simulink model "mainModel"  (R2024b)
settings: Solver=ode4  StartTime=0.0  StopTime=35000  FixedStep=0.1  RelTol=1e-3
values from neighbouring files (symbols this model uses):
  actuators = actuatorsConfig()    [main.m]
  constant = constantsConfig()    [main.m]
  control = controlConfig(data)    [main.m]
  MEKF = estimationConfig(sensors,simOpt)    [main.m]
  pert = pertConfig()    [main.m]
  sensors = sensorsConfig()    [main.m]
undefined symbols (not defined in the file or in its folder): Ab0, data, DiscIntNeverNeededParam, init
libraries: matrix_library x38, simulink x10, aerolibutil x7, simulink_extras x6, sharedtransform x1, dspinverses x1, dspfdesign x1, dspstat3 x1
(part 1 of 3)
settings Model: SimulationMode=accelerator  Creator=ricca  LastModifiedBy=ricca

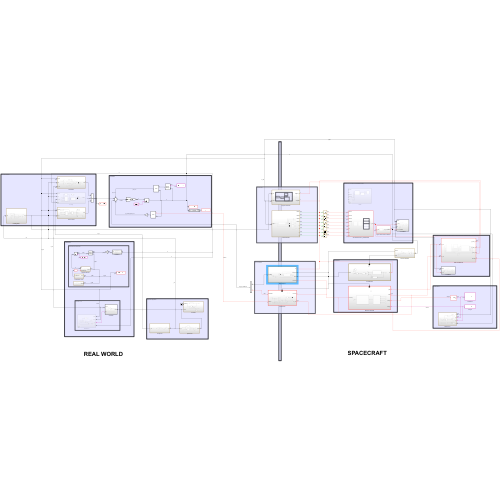
[thumbnail: Simulink's stored preview of the top-level diagram]
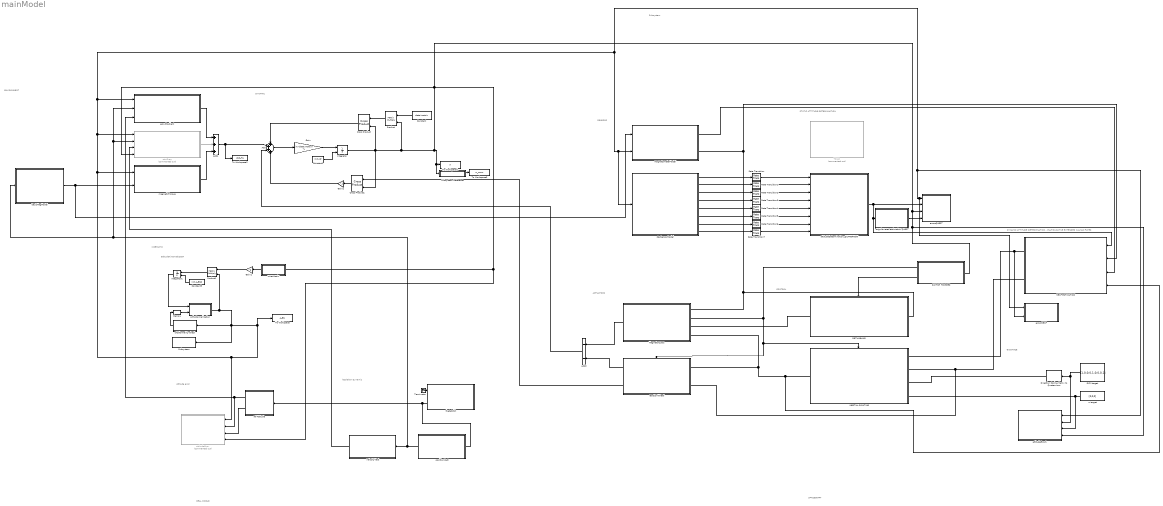
== system mainModel ==
  note: GUIDANCE
  note: DYNAMIC ATTITUDE DETERMINATION - MULTIPLICATIVE EXTENDED KALMAN FILTER
  note: SPACECRAFT
  note: REAL WORLD
  note: Subsystem
  note: ACTUATORS
  note: CONTROL
  note: STATIC ATTITUDE DETERMINATION
  note: SENSORS
  note: KINEMATIC
  note: Attitude error
  note: keplerian Dynamic
  note: attitudeKinematicDCM
  note: DYNAMIC
  note: ENVIRONMENT
  Add : Sum  Inputs=++++
  Add1 : Sum  Inputs=+++
  Add2 : Sum  Inputs=--
  Constant : Constant  Value=data.Imatrix
  Constant1 : Constant  Value=init.w0'
  Constant3 : Constant  Value=init.A_BN0
  Cross Product : matrix_library/Cross Product
  Cross Product1 : matrix_library/Cross Product
  DCM target : Constant  Value=[1,0,0;0,1,0;0,0,1]
  DETUMBLING : Subsystem
  Direction Cosine Matrix to Quaternions : sharedtransform/Direction Cosine Matrix  to Quaternions  aMode=0  action=None  tolerance=eps(2)
      settings: LibrarySourceBlock=|
      | aerolibtransform2/Direction Cosine Matrix
      | to Quaternions
  Gain : Gain  Gain=inv(data.Imatrix)  Multiplication=Matrix(K*u)
  Gain1 : Gain  Gain=-1
  Gain2 : Gain  Gain=-1
  INERTIAL POINTING : Subsystem
  Integrator : Integrator  InitialConditionSource=external  InitialCondition=init.w0
  Integrator1 : Integrator  InitialConditionSource=external  InitialCondition=Ab0
  MEKF ESTIMATION : Subsystem
  Magnetorquers : Subsystem
  Memory : Memory  InheritSampleTime=on
  Product : Product  Multiplication=Matrix(*)
  Product1 : Product  Inputs=**  Multiplication=Matrix(*)
  Rate Transition{,1..7} (8 alike) : RateTransition  OutPortSampleTime=0.1
  SWITCH TRIGGER : Subsystem
  Subsystem : Subsystem
  Subsystem Reference : Subsystem  ReferencedSubsystem=vecNorm
  TRIAD : Subsystem  Commented=on
  Terminator : Terminator
  To Workspace : ToWorkspace  VariableName=A_BN  SampleTime=-1
  To Workspace1 : ToWorkspace  VariableName=w  SampleTime=-1
  To Workspace2 : ToWorkspace  VariableName=dist_Tq  SampleTime=-1
  To Workspace3 : ToWorkspace  VariableName=w_norm  SampleTime=-1
  "angular rates estimation QUEST " : Subsystem
  atmDrag : Subsystem  Commented=on
  attitudeDetermination_QUATERNION : Subsystem
  attitudeError : Subsystem  Commented=on
  attitudeError1 : Subsystem
  basicMagModel : Subsystem
  errorsMEKF : Subsystem
  errorsQUEST : Subsystem
  gravGradient : Subsystem
  magneticTorque : Subsystem
  magnetometerModel : Subsystem
  orthoNormalization : Subsystem
  ortoNormality-check : Subsystem
  positionVect : Subsystem
  reactionWheel : Subsystem
  ref Attitude : Subsystem
  starSensorModel : Subsystem
  thetaOrbit : Subsystem
  velocityVect : Subsystem
  w target : Constant  Value=[0,0,0]
  wHatMatrix : Subsystem
  wires:
  Add/1 -> Gain/1  "M_TOT"
  Constant/1 -> Product/1
  Cross Product/1 -> Add/1  "(I*w) x w"
  Product/1 -> Cross Product/1
  Gain/1 -> Integrator/1
  Add1/1 -> Add/2, To Workspace2/1  "M_PERTURBATIONS"
  Constant1/1 -> Integrator/2
  gravGradient/1(GG) -> Add1/1
  basicMagModel/1(b_N) -> magnetometerModel/1(b_N), magneticTorque/2(b_N)
  orthoNormalization/1(Anew) -> Product1/2, ortoNormality-check/1(Anew), Subsystem/1(Anew), To Workspace/1, magnetometerModel/2(A_BN), starSensorModel/1(A_BN), attitudeError1/1(A), errorsMEKF/1(Anew), errorsQUEST/1(Anew), gravGradient/1(A_BN), atmDrag/1(A_BN), magneticTorque/1(A_BN), attitudeError/1(A_BN)  "A_BN"
  Gain1/1 -> Product1/1
  Product1/1 -> Integrator1/1  "Adot"
  Integrator1/1 -> orthoNormalization/1(A)  "A"
  wHatMatrix/1("[w]") -> Gain1/1
  Constant3/1 -> Integrator1/2
  Cross Product1/1 -> Gain2/1
  Integrator/1 -> Cross Product1/2, errorsQUEST/3(w), SWITCH TRIGGER/1(w), attitudeError1/4(w), wHatMatrix/1(w), attitudeError/4(w), atmDrag/4(w_B), Subsystem Reference/1, To Workspace1/1, Product/2, Cross Product/2  "w"
  positionVect/1(r_N) -> basicMagModel/1(r_N), gravGradient/2(r_N), atmDrag/2(r_N), velocityVect/1(r_N)  "r_N"
  thetaOrbit/2(theta) -> positionVect/1(theta), ref Attitude/1(theta)
  thetaOrbit/1(thetaDot) -> Terminator/1
  ref Attitude/2(w_L) -> attitudeError/3(w_L)
  ref Attitude/1(A_LN) -> gravGradient/3(A_LN), attitudeError/2(A_LN)  "A_LN"
  velocityVect/1(v_N) -> atmDrag/3(vel_N)  "vel_N"
  atmDrag/1(DRAG) -> Add1/2
  Memory/1 -> orthoNormalization/2(errOrtNormA)
  ortoNormality-check/1(errOrtNormA) -> Memory/1
  magneticTorque/1(MT) -> Add1/3
  attitudeDetermination_QUATERNION/1(q_est) -> MEKF ESTIMATION/1(q_meas_in), "angular rates estimation QUEST "/1(q_est), errorsQUEST/2(q_est)
  "angular rates estimation QUEST "/1(w_est_QUEST) -> errorsQUEST/4(w_est_QUEST)
  starSensorModel/1(sMeas1) -> Rate Transition/1
  starSensorModel/2(sMeas2) -> Rate Transition1/1
  starSensorModel/3(sMeas3) -> Rate Transition2/1
  starSensorModel/4(sMeas4) -> Rate Transition3/1
  starSensorModel/5(r1) -> Rate Transition4/1
  starSensorModel/6(r2) -> Rate Transition5/1
  starSensorModel/7(r3) -> Rate Transition6/1
  starSensorModel/8(r4) -> Rate Transition7/1
  Rate Transition/1 -> attitudeDetermination_QUATERNION/1(sMeas1)
  Rate Transition1/1 -> attitudeDetermination_QUATERNION/2(sMeas2)
  Rate Transition2/1 -> attitudeDetermination_QUATERNION/3(sMeas3)
  Rate Transition3/1 -> attitudeDetermination_QUATERNION/4(sMeas4)
  Rate Transition4/1 -> attitudeDetermination_QUATERNION/5(r1)
  Rate Transition5/1 -> attitudeDetermination_QUATERNION/6(r2)
  Rate Transition6/1 -> attitudeDetermination_QUATERNION/7(r3)
  Rate Transition7/1 -> attitudeDetermination_QUATERNION/8(r4)
  magnetometerModel/1(magReal_N) -> MEKF ESTIMATION/3(b_real_N)
  magnetometerModel/2(magMeas) -> MEKF ESTIMATION/2(b_meas_B), Magnetorquers/1(B), DETUMBLING/1(B)
  DCM target/1 -> Direction Cosine Matrix to Quaternions/1, attitudeError1/2(A_t)
  MEKF ESTIMATION/1(q_corr) -> errorsMEKF/2(q_corr), INERTIAL POINTING/1(qEst)  "qEst"
  MEKF ESTIMATION/2(w_corr) -> reactionWheel/2(w_corr), INERTIAL POINTING/2(wEst)  "wEst"
  Direction Cosine Matrix to Quaternions/1 -> INERTIAL POINTING/3(qTarget)  "qTarget"
  w target/1 -> attitudeError1/3(w_t), INERTIAL POINTING/4(wTarget)  "wTarget"
  DETUMBLING/1(mDet) -> Magnetorquers/3(mDet)
  INERTIAL POINTING/1(controlTq) -> MEKF ESTIMATION/4(controlTq), Magnetorquers/4(controlTq), reactionWheel/1(controlTq)
  Magnetorquers/1(magEffTq) -> Add2/1
  reactionWheel/1(hDotWheel) -> Add2/2  "hDot"
  reactionWheel/2(hWheel) -> Cross Product1/1  "hWheel"
  Gain2/1 -> Add/4  "-(I_wheel*w_wheel) x w"
  Add2/1 -> Add/3  "magTq - hDotWheel"
  SWITCH TRIGGER/1(isPoint) -> reactionWheel/Enable, INERTIAL POINTING/Enable, Magnetorquers/2(det2point)
  SWITCH TRIGGER/2(isDet) -> DETUMBLING/Enable
  Subsystem Reference/1 -> To Workspace3/1

== system mainModel/DETUMBLING ==
  B : Inport
  Enable : EnablePort
  Divide : Product  Inputs=*/
  Gain : Gain  Gain=-control.Kdet
  Saturation : Saturate  UpperLimit=actuators.magTorq.maxDipole  LowerLimit=-actuators.magTorq.maxDipole
  Scope : Scope
  Subsystem Reference : Subsystem  ReferencedSubsystem=vecNorm
  Terminator : Terminator
  compute Bdot : Subsystem
  mDet : Outport
  wires:
  B/1 -> Subsystem Reference/1, compute Bdot/1(B)
  Subsystem Reference/2 -> Terminator/1
  compute Bdot/1(Bdot) -> Divide/1
  Subsystem Reference/1 -> Divide/2
  Divide/1 -> Gain/1
  Gain/1 -> Saturation/1
  Saturation/1 -> Scope/1, mDet/1

== system mainModel/INERTIAL POINTING ==
  qEst : Inport
  wEst : Inport  Port=2
  qTarget : Inport  Port=3
  wTarget : Inport  Port=4
  Enable : EnablePort
  Define Error State : Subsystem
  PD conroller : Subsystem
  controlTq : Outport
  wires:
  Define Error State/1(alphaState) -> PD conroller/1(alphaState)
  qTarget/1 -> Define Error State/3(qTarget)
  wTarget/1 -> Define Error State/4(wTarget)
  qEst/1 -> Define Error State/1(qEst)
  PD conroller/1(controlTq) -> controlTq/1
  wEst/1 -> Define Error State/2(wEst)

== system mainModel/MEKF ESTIMATION ==
  q_meas_in : Inport
  b_meas_B : Inport  Port=2
  b_real_N : Inport  Port=3
  controlTq : Inport  Port=4
  CORRECTION : Subsystem
  Constant{,4..6} (4 alike) : Constant  Value=[0,0,0]
  Constant2 : Constant  Value=data.Imatrix
  MEASUREMENT : Subsystem
  Memory : Memory  InitialCondition=MEKF.init.P
  Memory1 : Memory  InitialCondition=MEKF.init.w
  Memory2 : Memory  InitialCondition=MEKF.init.q
  PREDICTION : Subsystem
  Scope : Scope
  q_corr : Outport
  w_corr : Outport  Port=2
  wires:
  Constant2/1 -> PREDICTION/4(J)
  CORRECTION/3(P_corr) -> Memory/1
  CORRECTION/2(w_corr) -> Memory1/1
  CORRECTION/1(q_corr) -> Memory2/1
  Memory/1 -> PREDICTION/3(P_corr)  "P_corr"
  Memory2/1 -> Scope/1, q_corr/1, PREDICTION/1(q_corr)  "q_corr"
  Memory1/1 -> w_corr/1, PREDICTION/2(w_corr)  "w_corr"
  Constant/1 -> PREDICTION/5(distTq)
  Constant4/1 -> ?
  Constant5/1 -> PREDICTION/7(hWheel)
  Constant6/1 -> PREDICTION/8(hDotWheel)
  MEASUREMENT/1(y) -> CORRECTION/1(y)
  MEASUREMENT/2(K) -> CORRECTION/2(K)
  MEASUREMENT/3(H) -> CORRECTION/3(H)
  PREDICTION/1(q_pred) -> MEASUREMENT/4(q_pred), CORRECTION/4(q_pred)
  PREDICTION/3(P_pred) -> MEASUREMENT/5(P_pred), CORRECTION/6(P_pred)
  b_real_N/1 -> MEASUREMENT/3(b_real_N)
  b_meas_B/1 -> MEASUREMENT/2(b_meas_B)
  q_meas_in/1 -> MEASUREMENT/1(q_meas_in)
  PREDICTION/2(w_pred) -> CORRECTION/5(w_pred)
  controlTq/1 -> PREDICTION/6(controlTq)

== system mainModel/Magnetorquers ==
  B : Inport
  det2point : Inport  Port=2
  mDet : Inport  Port=3
  controlTq : Inport  Port=4
  Band-Limited White Noise : simulink/Sources/Band-Limited White Noise  Cov=1e-12  Ts=0.1  seed=[23341]
  Cross Product : matrix_library/Cross Product
  Merge : Merge
  Quantizer : Quantizer  QuantizationInterval=1e-8
  Scope : Scope
  Subsystem : Subsystem
  Sum : Sum  Inputs=|++
  To Workspace : ToWorkspace  VariableName=magEffTorque  SampleTime=-1
  To Workspace1 : ToWorkspace  VariableName=magDipole  SampleTime=-1
  magEffTq : Outport
  wires:
  Cross Product/1 -> Sum/1
  B/1 -> Cross Product/2, Subsystem/2(B)  "B"
  Sum/1 -> To Workspace/1, magEffTq/1
  controlTq/1 -> Quantizer/1
  Subsystem/1(m) -> Merge/2
  Merge/1 -> Scope/1, To Workspace1/1, Cross Product/1  "m"
  mDet/1 -> Merge/1
  det2point/1 -> Subsystem/Enable
  Band-Limited White Noise/1 -> Sum/2
  Quantizer/1 -> Subsystem/1(controlTq)

== system mainModel/SWITCH TRIGGER ==
  w : Inport
  Add : Sum
  Cast To Single : DataTypeConversion  OutDataTypeStr=single  SaturateOnIntegerOverflow=off  RndMeth=Floor
  Compare To Constant : simulink/Logic and Bit Operations/Compare To Constant  relop=<=  const=data.detumb.wNormMin  OutDataTypeStr=boolean
  Compare To Constant1 : simulink/Logic and Bit Operations/Compare To Constant  relop=>=  const=100  OutDataTypeStr=boolean
  Memory : Memory  InheritSampleTime=on
  NOT : Logic  Operator=NOT  AllPortsSameDT=off  OutDataTypeStr=boolean
  Scope : Scope
  Scope1 : Scope
  Scope5 : Scope
  Subsystem Reference : Subsystem  ReferencedSubsystem=vecNorm
  Terminator : Terminator
  To Workspace : ToWorkspace  VariableName=enablePoint  SampleTime=-1
  isPoint : Outport
  isDet : Outport  Port=2
  wires:
  w/1 -> Scope1/1, Subsystem Reference/1
  Subsystem Reference/1 -> Scope5/1, Compare To Constant/1
  Subsystem Reference/2 -> Terminator/1
  Compare To Constant/1 -> Cast To Single/1
  Memory/1 -> Add/1
  Add/1 -> Memory/1, Compare To Constant1/1
  Cast To Single/1 -> Add/2
  Compare To Constant1/1 -> NOT/1, isPoint/1, Scope/1
  NOT/1 -> To Workspace/1, isDet/1

== system mainModel/Subsystem ==
  Anew : Inport
  Constant : Constant
  Cross Product : matrix_library/Cross Product
  Dot Product : DotProduct  OutDataTypeStr=Inherit: Inherit via internal rule
  Minus : Sum  Inputs=+-
  Scope : Scope
  Selector : Selector  NumberOfDimensions=2  InputPortWidth=3  IndexOptions=Select all,Index vector (dialog)  Indices=[1 3],1  OutputSizes=1,1
  Selector1 : Selector  NumberOfDimensions=2  InputPortWidth=3  IndexOptions=Select all,Index vector (dialog)  Indices=[1 3],2  OutputSizes=1,1
  Selector2 : Selector  NumberOfDimensions=2  InputPortWidth=3  IndexOptions=Select all,Index vector (dialog)  Indices=[1 3],3  OutputSizes=1,1
  To Workspace : ToWorkspace  VariableName=rightHandleCheck  SampleTime=-1
  wires:
  Anew/1 -> Selector/1, Selector2/1, Selector1/1
  Selector/1 -> Cross Product/1
  Selector1/1 -> Cross Product/2
  Cross Product/1 -> Dot Product/1
  Selector2/1 -> Dot Product/2
  Constant/1 -> Minus/2
  Dot Product/1 -> Minus/1
  Minus/1 -> Scope/1, To Workspace/1

== system mainModel/TRIAD ==
  A_BN : Inport
  w : Inport  Port=2
  sMeas1 : Inport  Port=3
  sMeas2 : Inport  Port=4
  r1 : Inport  Port=5
  r2 : Inport  Port=6
  "angular rates estimation TRIAD " : Subsystem
  attitudeDetermination_TRIAD : Subsystem
  errorsTRIAD : Subsystem
  wires:
  attitudeDetermination_TRIAD/1(A_BN_est) -> "angular rates estimation TRIAD "/1(A_BN_est), errorsTRIAD/2(A_BN_est)
  sMeas1/1 -> attitudeDetermination_TRIAD/1(sMeas1)
  w/1 -> errorsTRIAD/3(w)
  sMeas2/1 -> attitudeDetermination_TRIAD/2(sMeas2)
  r1/1 -> attitudeDetermination_TRIAD/3(r1)
  "angular rates estimation TRIAD "/1(w_estTRIAD) -> errorsTRIAD/4(w_estTRIAD)
  A_BN/1 -> errorsTRIAD/1(A_BN)
  r2/1 -> attitudeDetermination_TRIAD/4(r2)

== system mainModel/angular rates estimation QUEST  ==
  q_est : Inport
  To Workspace1 : ToWorkspace  VariableName=w_est_QUEST  SampleTime=-1
  angVelEstimation : Subsystem
  svd : Subsystem  Commented=on
  w_est_QUEST : Outport
  wires:
  angVelEstimation/1(w_est) -> w_est_QUEST/1, To Workspace1/1
  q_est/1 -> angVelEstimation/1(q_est)

== system mainModel/atmDrag ==
  A_BN : Inport
  r_N : Inport  Port=2
  vel_N : Inport  Port=3
  w_B : Inport  Port=4
  "DRAG torque " : Subsystem
  Reshape : Reshape
  Scope : Scope
  To Workspace : ToWorkspace  VariableName=dragPert  SampleTime=-1
  density : Subsystem
  relVel : Subsystem
  trash : Subsystem  Commented=on  TreatAsAtomicUnit=on
  DRAG : Outport
  wires:
  A_BN/1 -> relVel/1(A_BN)
  r_N/1 -> density/1(r_N), relVel/2(r_N)
  vel_N/1 -> relVel/3(vel_N)
  relVel/1(velRel_B) -> "DRAG torque "/2(velRel_B)
  density/1(rho) -> "DRAG torque "/1(rho)
  w_B/1 -> "DRAG torque "/3(w_B)
  "DRAG torque "/1(DRAG) -> Reshape/1
  Reshape/1 -> Scope/1, To Workspace/1, DRAG/1

== system mainModel/attitudeDetermination_QUATERNION ==
  note: QUEST - SHUSTER
  note: DAVENPORT'S q-METHOD (MAT FUNC)
  note: QUEST METHOD
  sMeas1 : Inport
  sMeas2 : Inport  Port=2
  sMeas3 : Inport  Port=3
  sMeas4 : Inport  Port=4
  r1 : Inport  Port=5
  r2 : Inport  Port=6
  r3 : Inport  Port=7
  r4 : Inport  Port=8
  QUEST : Subsystem
  QUEST V2 : Subsystem
  Scope : Scope
  Terminator{,1..3} (4 alike) : Terminator
  compute Bmatrix : Subsystem
  compute Kmatrix : Subsystem
  matlaFunction for Davenport's q-method : Subsystem
  quest - shuster : Subsystem
  q_est : Outport
  wires:
  sMeas1/1 -> compute Bmatrix/1(s1)  "s1"
  sMeas2/1 -> compute Bmatrix/2(s2)  "s2"
  sMeas3/1 -> compute Bmatrix/3(s3)  "s3"
  r1/1 -> compute Bmatrix/5(v1)  "v1"
  r2/1 -> compute Bmatrix/6(v2)  "v2"
  r3/1 -> compute Bmatrix/7(v3)  "v3"
  compute Bmatrix/1(B) -> compute Kmatrix/1(B)
  compute Kmatrix/2(S) -> QUEST V2/3(S), QUEST/1(S), quest - shuster/1(S)
  compute Kmatrix/4(sigma) -> QUEST/3(sigma), QUEST V2/2(sigma)
  matlaFunction for Davenport's q-method/1(q_est) -> q_est/1
  r4/1 -> compute Bmatrix/8(v4)  "v4"
  sMeas4/1 -> compute Bmatrix/4(s4)  "s4"
  compute Kmatrix/3(z) -> QUEST/2(z), QUEST V2/1(z), quest - shuster/2(z)
  compute Kmatrix/1(K) -> matlaFunction for Davenport's q-method/1(K)
  matlaFunction for Davenport's q-method/2(lambda_max) -> Scope/1
  QUEST V2/1(q_est) -> Terminator1/1
  QUEST/1(q_est) -> Terminator/1
  quest - shuster/1(q_est) -> Terminator2/1
  quest - shuster/2(lambda) -> Terminator3/1

== system mainModel/attitudeError ==
  note: w_BL
  note: attitudeError
  A_BN : Inport
  A_LN : Inport  Port=2
  w_L : Inport  Port=3
  w : Inport  Port=4
  A_BL * w_L : Product  Multiplication=Matrix(*)
  A_BN * A_LN^t : Product  Multiplication=Matrix(*)
  Minus : Sum  Inputs=-+
  Scope1 : Scope
  Scope2 : Scope
  Scope4 : Scope
  To Workspace : ToWorkspace  VariableName=A_BL  SampleTime=-1
  To Workspace1 : ToWorkspace  VariableName=angVelError  SampleTime=-1
  Transpose : Math  Operator=transpose
  angle error : Subsystem
  wires:
  A_LN/1 -> Transpose/1
  A_BN/1 -> angle error/1(Aerr), A_BN * A_LN^t/1
  Transpose/1 -> A_BN * A_LN^t/2
  A_BN * A_LN^t/1 -> To Workspace/1, Scope1/1, A_BL * w_L/1  "A_BL"
  w_L/1 -> A_BL * w_L/2
  A_BL * w_L/1 -> Minus/1
  w/1 -> Minus/2
  Minus/1 -> To Workspace1/1, Scope2/1  "angVelError"
  angle error/1(theta_err) -> Scope4/1

== system mainModel/attitudeError1 ==
  A : Inport
  A_t : Inport  Port=2
  w_t : Inport  Port=3
  w : Inport  Port=4
  A_s * A_t^t : Product  Multiplication=Matrix(*)
  Minus : Sum  Inputs=-+
  Scope1 : Scope
  Scope2 : Scope
  Scope4 : Scope
  To Workspace : ToWorkspace  VariableName=A_err  SampleTime=-1
  To Workspace1 : ToWorkspace  VariableName=wError  SampleTime=-1
  To Workspace2 : ToWorkspace  VariableName=thetaErr  SampleTime=-1
  Transpose : Math  Operator=transpose
  angle error : Subsystem
  wires:
  A_t/1 -> Transpose/1
  A/1 -> angle error/1(Aerr), A_s * A_t^t/1
  Transpose/1 -> A_s * A_t^t/2
  A_s * A_t^t/1 -> To Workspace/1, Scope1/1  "A_e"
  w/1 -> Minus/2
  Minus/1 -> To Workspace1/1, Scope2/1  "wError"
  angle error/1(theta_err) -> Scope4/1, To Workspace2/1
  w_t/1 -> Minus/1

== system mainModel/basicMagModel ==
  r_N : Inport
  Add : Sum  Inputs=+-
  Constant : Constant  Value=pert.mf.H0
  Constant1 : Constant  Value=3
  Constant2 : Constant  Value=3
  Constant3 : Constant  Value=constant.Re
  Constant4 : Constant  Value=constant.we
  Constant5 : Constant  Value=pert.mf.magAxAngle
  Divide : Product  Inputs=/*
  Gain : Gain  Gain=3
  Power1 : Math  Operator=pow
  Power2 : Math  Operator=pow
  Product : Product
  Product1 : Product
  Product2 : Product
  Scope : Scope
  Subsystem Reference : Subsystem  ReferencedSubsystem=vecNorm
      settings: PortSchema="{\"entries\":[{\"content\":{\"sides\":[{\"content\":{\"connectorIds\":[\"In1\"]},\"type\":\"ConnectorPlacement.EquallySpacedRectSide\",\"uuid\":\"3c656289-fd98-4ca2-a1ed-c6410d06bb5d\"},{\"content\":{\"connectorIds\":[\"Out2\",\"Out1\"],\"side\":\"RIGHT\"},\"type\":\"ConnectorPlacement.EquallySpacedRectSide\",\"uuid\":\"08457cd9-a03f-41e7-acb1-b2e1b3c4ce0a\"},{\"content\":{\"side\":\"TOP\"},\"type\":\"ConnectorPlacement.EquallySpacedRectSide\",\"uuid\":\"d406813d-879a-4017-a475-3b86ba09a3ff\"}]},\"type\":\"ConnectorPlacement.EquallySpacedConnector\",\"uuid\":\"69498d47-a241-4b2e-9db5-57ee60b53d10\"}],\"packageUris\":[\"http://schema.mathworks.com/mf0/Connector/R2020b\"],\"version\":\"1.0\"}"
  To Workspace : ToWorkspace  VariableName=b_N  SampleTime=-1
  m dot r : DotProduct  OutDataTypeStr=Inherit: Inherit via internal rule
  mHat : Subsystem
  b_N : Outport
  wires:
  Constant1/1 -> Power1/2
  Constant4/1 -> mHat/1(we)
  Power1/1 -> Product/1
  Constant/1 -> Product/2
  Product/1 -> Divide/2
  mHat/1(mHat) -> m dot r/1, Add/2
  m dot r/1 -> Product1/2
  Product1/1 -> Gain/1
  Gain/1 -> Add/1
  Add/1 -> Product2/2
  Divide/1 -> Product2/1
  Product2/1 -> b_N/1, To Workspace/1, Scope/1
  Constant2/1 -> Power2/2
  Power2/1 -> Divide/1
  Subsystem Reference/1 -> Power2/1
  Subsystem Reference/2 -> m dot r/2, Product1/1  "r_vers"
  r_N/1 -> Subsystem Reference/1
  Constant3/1 -> Power1/1
  Constant5/1 -> mHat/2(magAxAngle)

== system mainModel/errorsMEKF ==
  Anew : Inport
  q_corr : Inport  Port=2
  Demux : Demux
  Mux : Mux
  Scope{1..2,4..5} (4 alike) : Scope
  TRUE^t * SYM : Product  Multiplication=Matrix(*)
  To Workspace : ToWorkspace  VariableName=thetaErrMekf  SampleTime=-1
  Transpose : Math  Operator=transpose
  Zero-Order Hold1 : ZeroOrderHold  SampleTime=0.1
  angle error : Subsystem
  quat2DCM : Subsystem  ReferencedSubsystem=quat2DCM
  wires:
  q_corr/1 -> Demux/1
  Anew/1 -> Zero-Order Hold1/1
  angle error/1(theta_err) -> To Workspace/1, Scope4/1  "errMEKF"
  TRUE^t * SYM/1 -> Scope5/1, angle error/1(Aerr)
  quat2DCM/1 -> Scope1/1, TRUE^t * SYM/2
  Zero-Order Hold1/1 -> Scope2/1, Transpose/1
  Transpose/1 -> TRUE^t * SYM/1
  Demux/1 -> Mux/4
  Demux/2 -> Mux/1
  Demux/3 -> Mux/2
  Demux/4 -> Mux/3
  Mux/1 -> quat2DCM/1

== system mainModel/errorsQUEST ==
  Anew : Inport
  q_est : Inport  Port=2
  w : Inport  Port=3
  w_est_QUEST : Inport  Port=4
  Minus : Sum  Inputs=+-
  Scope{,1..2,4..5} (5 alike) : Scope
  Scope3 : Scope  NumInputPorts=2
  TRUE^t * SYM : Product  Multiplication=Matrix(*)
  To Workspace : ToWorkspace  VariableName=thetaErrQ  SampleTime=-1
  Transpose : Math  Operator=transpose
  Zero-Order Hold : ZeroOrderHold  SampleTime=0.1
  Zero-Order Hold1 : ZeroOrderHold  SampleTime=0.1
  angle error : Subsystem
  quat2DCM : Subsystem  ReferencedSubsystem=quat2DCM
  wires:
  w_est_QUEST/1 -> Scope3/2, Minus/1
  w/1 -> Zero-Order Hold/1
  Minus/1 -> Scope/1
  q_est/1 -> quat2DCM/1
  Anew/1 -> Zero-Order Hold1/1
  Transpose/1 -> TRUE^t * SYM/1
  TRUE^t * SYM/1 -> Scope5/1, angle error/1(Aerr)
  quat2DCM/1 -> Scope1/1, TRUE^t * SYM/2
  angle error/1(theta_err) -> To Workspace/1, Scope4/1  "errQUEST"
  Zero-Order Hold/1 -> Scope3/1, Minus/2
  Zero-Order Hold1/1 -> Scope2/1, Transpose/1

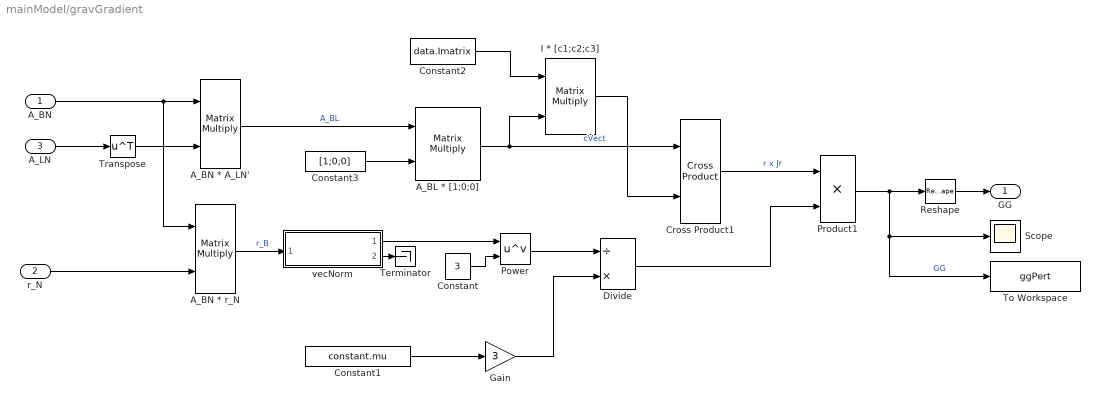
== system mainModel/gravGradient ==
  A_BN : Inport
  r_N : Inport  Port=2
  A_LN : Inport  Port=3
  A_BL * [1;0;0] : Product  Multiplication=Matrix(*)
  A_BN * A_LN' : Product  Multiplication=Matrix(*)
  A_BN * r_N : Product  Multiplication=Matrix(*)
  Constant : Constant  Value=3
  Constant1 : Constant  Value=constant.mu
  Constant2 : Constant  Value=data.Imatrix
  Constant3 : Constant  Value=[1;0;0]
  Cross Product1 : matrix_library/Cross Product
  Divide : Product  Inputs=/*
  Gain : Gain  Gain=3
  I * [c1;c2;c3] : Product  Multiplication=Matrix(*)
  Power : Math  Operator=pow
  Product1 : Product
  Reshape : Reshape
  Scope : Scope
  Terminator : Terminator
  To Workspace : ToWorkspace  VariableName=ggPert  SampleTime=-1
  Transpose : Math  Operator=transpose
  vecNorm : Subsystem  ReferencedSubsystem=vecNorm
  GG : Outport
  wires:
  Constant3/1 -> A_BL * [1;0;0]/2
  A_BN * A_LN'/1 -> A_BL * [1;0;0]/1  "A_BL"
  A_BL * [1;0;0]/1 -> Cross Product1/1, I * [c1;c2;c3]/2  "cVect"
  Product1/1 -> Reshape/1, To Workspace/1, Scope/1  "GG"
  Transpose/1 -> A_BN * A_LN'/2
  A_BN/1 -> A_BN * A_LN'/1, A_BN * r_N/1
  A_LN/1 -> Transpose/1
  Divide/1 -> Product1/2
  Power/1 -> Divide/1
  Constant/1 -> Power/2
  r_N/1 -> A_BN * r_N/2
  A_BN * r_N/1 -> vecNorm/1  "r_B"
  Constant1/1 -> Gain/1
  Gain/1 -> Divide/2
  vecNorm/2 -> Terminator/1
  I * [c1;c2;c3]/1 -> Cross Product1/2
  Constant2/1 -> I * [c1;c2;c3]/1
  Cross Product1/1 -> Product1/1  "r x Jr"
  Reshape/1 -> GG/1
  vecNorm/1 -> Power/1

== system mainModel/magneticTorque ==
  A_BN : Inport
  b_N : Inport  Port=2
  A_BN * b_N : Product  Multiplication=Matrix(*)
  Constant : Constant  Value=pert.mf.j_B
  Scope : Scope
  To Workspace : ToWorkspace  VariableName=magFPert  SampleTime=-1
  j_B x b_B : matrix_library/Cross Product
  MT : Outport
  wires:
  A_BN/1 -> A_BN * b_N/1
  A_BN * b_N/1 -> j_B x b_B/2  "b_B"
  Constant/1 -> j_B x b_B/1
  j_B x b_B/1 -> To Workspace/1, MT/1, Scope/1  "MT"
  b_N/1 -> A_BN * b_N/2

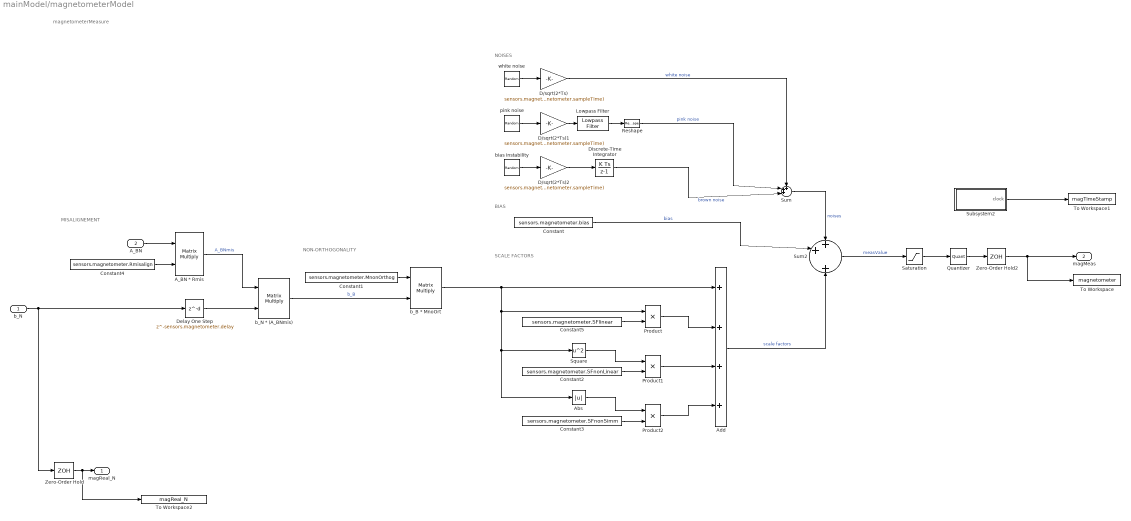
== system mainModel/magnetometerModel ==
  note: SCALE FACTORS
  note: magnetometerMeasure
  note: NON-ORTHOGONALITY
  note: NOISES
  note: BIAS
  note: MISALIGNEMENT
  b_N : Inport
  A_BN : Inport  Port=2
  A_BN * Rmis : Product  Multiplication=Matrix(*)
  Abs : Abs  SaturateOnIntegerOverflow=off
  Add : Sum  Inputs=++++
  Constant : Constant  Value=sensors.magnetometer.bias
  Constant1 : Constant  Value=sensors.magnetometer.MnonOrthog
  Constant2 : Constant  Value=sensors.magnetometer.SFnonLinear
  Constant3 : Constant  Value=sensors.magnetometer.SFnonSimm
  Constant4 : Constant  Value=sensors.magnetometer.Rmisalign
  Constant5 : Constant  Value=sensors.magnetometer.SFlinear
  D/sqrt(2*Ts) : Gain  Gain=sensors.magnetometer.noiseDensity/sqrt(2*sensors.magnetometer.sampleTime)
  D/sqrt(2*Ts)1 : Gain  Gain=sensors.magnetometer.noiseDensity/sqrt(2*sensors.magnetometer.sampleTime)
  D/sqrt(2*Ts)2 : Gain  Gain=sensors.magnetometer.noiseDensity/sqrt(2*sensors.magnetometer.sampleTime)
  Delay One Step : Delay  DelayLength=sensors.magnetometer.delay
  Discrete-Time Integrator : DiscreteIntegrator  SampleTime=-1  ICPrevOutput=DiscIntNeverNeededParam  ICPrevScaledInput=DiscIntNeverNeededParam
  Lowpass Filter : dspfdesign/Lowpass Filter  FilterType=FIR  DesignForMinimumOrder=on  FilterOrder=50  PassbandFrequency=0.01  StopbandFrequency=0.99  PassbandRipple=0.1  StopbandAttenuation=80  SampleRateMode=Use normalized frequency (0 to 1)  SampleRate=44100  SimulateUsing=Interpreted execution  roundingMode=Floor  coeffsDataTypeStr=fixdt(1,16)
  Product : Product
  Product1 : Product
  Product2 : Product
  Quantizer : Quantizer  QuantizationInterval=sensors.magnetometer.resolution
  Reshape : Reshape
  Saturation : Saturate  UpperLimit=sensors.magnetometer.saturation  LowerLimit=-sensors.magnetometer.saturation
  Square : Math  Operator=square
  Subsystem2 : Subsystem
  Sum : Sum  Inputs=+++|
  Sum2 : Sum  Inputs=++|+
  To Workspace : ToWorkspace  VariableName=magnetometer  SaveFormat=Structure With Time  SampleTime=-1
  To Workspace1 : ToWorkspace  VariableName=magTimeStamp  SaveFormat=Structure With Time  SampleTime=-1
  To Workspace2 : ToWorkspace  VariableName=magReal_N  SampleTime=-1
  Zero-Order Hold : ZeroOrderHold  SampleTime=sensors.magnetometer.sampleTime
  Zero-Order Hold2 : ZeroOrderHold  SampleTime=sensors.magnetometer.sampleTime
  b_B * MnoOrt : Product  Multiplication=Matrix(*)
  b_N * (A_BNmis) : Product  Multiplication=Matrix(*)
  bias instability : RandomNumber  Seed=sensors.magnetometer.noiseSeed  SampleTime=0.1
  pink noise : RandomNumber  Seed=sensors.magnetometer.noiseSeed  SampleTime=0.1
  white noise : RandomNumber  Seed=sensors.magnetometer.noiseSeed  SampleTime=0.1
  magReal_N : Outport
  magMeas : Outport  Port=2
  wires:
  Subsystem2/1(clock) -> To Workspace1/1
  A_BN/1 -> A_BN * Rmis/1
  Sum/1 -> Sum2/1  "noises"
  Delay One Step/1 -> b_N * (A_BNmis)/2
  white noise/1 -> D/sqrt(2*Ts)/1
  pink noise/1 -> D/sqrt(2*Ts)1/1
  bias instability/1 -> D/sqrt(2*Ts)2/1
  D/sqrt(2*Ts)1/1 -> Lowpass Filter/1
  D/sqrt(2*Ts)/1 -> Sum/1  "white noise"
  D/sqrt(2*Ts)2/1 -> Discrete-Time Integrator/1
  Discrete-Time Integrator/1 -> Sum/3  "brown noise"
  Sum2/1 -> Saturation/1  "measValue"
  Constant/1 -> Sum2/2  "bias"
  Reshape/1 -> Sum/2  "pink noise"
  Lowpass Filter/1 -> Reshape/1
  Constant4/1 -> A_BN * Rmis/2
  Saturation/1 -> Quantizer/1
  Quantizer/1 -> Zero-Order Hold2/1
  A_BN * Rmis/1 -> b_N * (A_BNmis)/1  "A_BNmis"
  b_N * (A_BNmis)/1 -> b_B * MnoOrt/2  "b_B"
  Constant1/1 -> b_B * MnoOrt/1
  b_B * MnoOrt/1 -> Abs/1, Square/1, Product/1, Add/1
  Add/1 -> Sum2/3  "scale factors"
  Constant3/1 -> Product2/2
  Abs/1 -> Product2/1
  Constant2/1 -> Product1/2
  Square/1 -> Product1/1
  Product/1 -> Add/2
  Product1/1 -> Add/3
  Product2/1 -> Add/4
  Constant5/1 -> Product/2
  b_N/1 -> Zero-Order Hold/1, Delay One Step/1
  Zero-Order Hold/1 -> To Workspace2/1, magReal_N/1
  Zero-Order Hold2/1 -> To Workspace/1, magMeas/1

== system mainModel/orthoNormalization ==
  A : Inport
  errOrtNormA : Inport  Port=2
  Compare To Constant : simulink/Logic and Bit Operations/Compare To Constant  relop=<=  const=1e-8  OutDataTypeStr=boolean
  Switch : Switch  Criteria=u2 > Threshold  SaturateOnIntegerOverflow=off  InputSameDT=off
  orthonormalization : Subsystem
  Anew : Outport
  wires:
  A/1 -> orthonormalization/1(A), Switch/1  "A"
  Compare To Constant/1 -> Switch/2
  errOrtNormA/1 -> Compare To Constant/1
  Switch/1 -> Anew/1
  orthonormalization/1(Anew) -> Switch/3  "Anew"

== system mainModel/ortoNormality-check ==
  Anew : Inport
  Add : Sum  Inputs=+-
  Add1 : Sum  Inputs=+-
  Constant : Constant  Value=eye(3)
  Constant1 : Constant  Value=2
  Constant2 : Constant  Value=eye(3)
  Constant3 : Constant  Value=2
  MatrixMultiply : Product  Multiplication=Matrix(*)
  MatrixMultiply1 : Product  Multiplication=Matrix(*)
  Max : MinMax  Function=max  Inputs=2
  Power : Math  Operator=pow
  Power1 : Math  Operator=pow
  Reshape : Reshape
  Reshape1 : Reshape
  Scope : Scope
  Sqrt : Sqrt
  Sqrt1 : Sqrt
  Sum of Elements : Sum  Inputs=+
  Sum of Elements1 : Sum  Inputs=+
  To Workspace : ToWorkspace  VariableName=errOrtNormA  SampleTime=-1
  Transpose : Math  Operator=transpose
  Transpose1 : Math  Operator=transpose
  errOrtNormA : Outport
  wires:
  Transpose/1 -> MatrixMultiply/1
  MatrixMultiply/1 -> Add/1
  Sum of Elements/1 -> Sqrt/1
  Power/1 -> Sum of Elements/1
  Sqrt/1 -> Max/1
  Add/1 -> Reshape/1
  Constant1/1 -> Power/2
  Reshape/1 -> Power/1
  Constant/1 -> Add/2
  Constant2/1 -> Add1/2
  Add1/1 -> Reshape1/1
  Power1/1 -> Sum of Elements1/1
  MatrixMultiply1/1 -> Add1/1
  Transpose1/1 -> MatrixMultiply1/2
  Constant3/1 -> Power1/2
  Reshape1/1 -> Power1/1
  Anew/1 -> Transpose/1, MatrixMultiply/2, MatrixMultiply1/1, Transpose1/1
  Sum of Elements1/1 -> Sqrt1/1
  Sqrt1/1 -> Max/2
  Max/1 -> errOrtNormA/1, Scope/1, To Workspace/1

== system mainModel/positionVect ==
  theta : Inport
  Constant : Constant  Value=data.i
  Product : Product
  To Workspace : ToWorkspace  VariableName=r_N  SampleTime=-1
  direction : Subsystem
  value : Subsystem
  r_N : Outport
  wires:
  theta/1 -> value/1(theta), direction/1(theta)  "theta"
  Constant/1 -> direction/2(i)  "i"
  value/1(r) -> Product/1
  direction/1(dir) -> Product/2
  Product/1 -> To Workspace/1, r_N/1

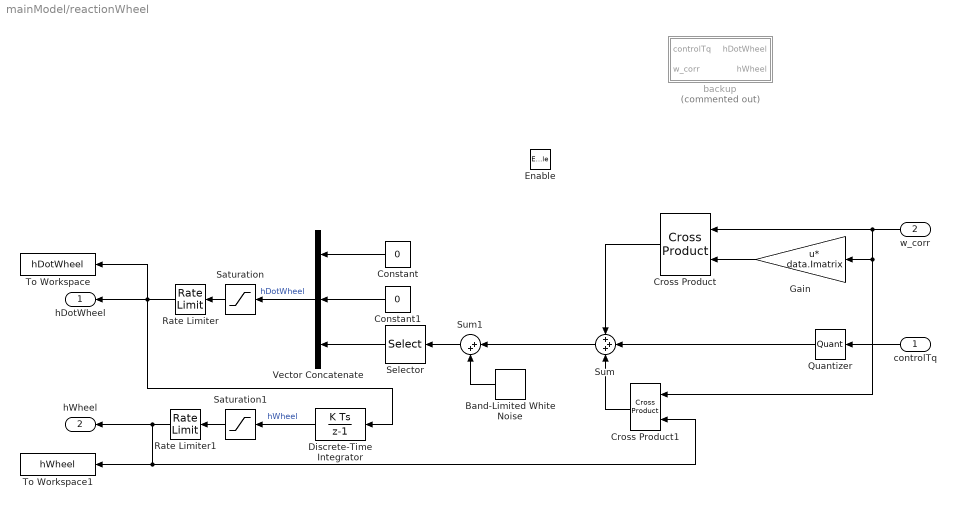
== system mainModel/reactionWheel ==
  controlTq : Inport
  w_corr : Inport  Port=2
  Enable : EnablePort
  Band-Limited White Noise : simulink/Sources/Band-Limited White Noise  Cov=[1e-12]  Ts=0.1  seed=[23341]
  Constant : Constant  Value=0
  Constant1 : Constant  Value=0
  Cross Product : matrix_library/Cross Product
  Cross Product1 : matrix_library/Cross Product
  Discrete-Time Integrator : DiscreteIntegrator  SampleTime=-1  LimitOutput=on  UpperSaturationLimit=actuators.wheel.maxMomentum  LowerSaturationLimit=-actuators.wheel.maxMomentum  ICPrevOutput=DiscIntNeverNeededParam  ICPrevScaledInput=DiscIntNeverNeededParam
  Gain : Gain  Gain=data.Imatrix  Multiplication=Matrix(u*K)
  Quantizer : Quantizer  QuantizationInterval=1e-6
  Rate Limiter : RateLimiter  RisingSlewLimit=actuators.wheel.maxSpeed  FallingSlewLimit=-actuators.wheel.maxSpeed  SampleTimeMode=inherited
  Rate Limiter1 : RateLimiter  RisingSlewLimit=actuators.wheel.maxSpeed  FallingSlewLimit=-actuators.wheel.maxSpeed  SampleTimeMode=inherited
  Saturation : Saturate  UpperLimit=actuators.wheel.maxTorque  LowerLimit=-actuators.wheel.maxTorque
  Saturation1 : Saturate  UpperLimit=actuators.wheel.maxMomentum  LowerLimit=-actuators.wheel.maxMomentum
  Selector : Selector  InputPortWidth=3  IndexOptions=Index vector (dialog)  Indices=3  OutputSizes=1
  Sum : Sum  Inputs=+++
  Sum1 : Sum  Inputs=|++
  To Workspace : ToWorkspace  VariableName=hDotWheel  SampleTime=-1
  To Workspace1 : ToWorkspace  VariableName=hWheel  SampleTime=-1
  Vector Concatenate : Concatenate  NumInputs=3
  backup : Subsystem  Commented=on
  hDotWheel : Outport
  hWheel : Outport  Port=2
  wires:
  controlTq/1 -> Quantizer/1
  Selector/1 -> Vector Concatenate/3
  Constant/1 -> Vector Concatenate/1
  Constant1/1 -> Vector Concatenate/2
  Vector Concatenate/1 -> Saturation/1  "hDotWheel"
  Discrete-Time Integrator/1 -> Saturation1/1  "hWheel"
  Sum/1 -> Sum1/1
  Rate Limiter1/1 -> To Workspace1/1, Cross Product1/2, hWheel/1
  Rate Limiter/1 -> To Workspace/1, hDotWheel/1, Discrete-Time Integrator/1
  Quantizer/1 -> Sum/2
  Band-Limited White Noise/1 -> Sum1/2
  Gain/1 -> Cross Product/2
  w_corr/1 -> Cross Product/1, Gain/1, Cross Product1/1
  Cross Product/1 -> Sum/1
  Cross Product1/1 -> Sum/3
  Saturation/1 -> Rate Limiter/1
  Saturation1/1 -> Rate Limiter1/1
  Sum1/1 -> Selector/1

== system mainModel/ref Attitude ==
  theta : Inport
  Constant : Constant  Value=data.wL
  R_theta * R_i : Product  Multiplication=Matrix(*)
  Subsystem : Subsystem
  Subsystem1 : Subsystem
  A_LN : Outport
  w_L : Outport  Port=2
  wires:
  Constant/1 -> w_L/1
  theta/1 -> Subsystem/1(theta)  "theta"
  R_theta * R_i/1 -> A_LN/1
  Subsystem/1(R_theta) -> R_theta * R_i/1
  Subsystem1/1(R_i) -> R_theta * R_i/2

== system mainModel/starSensorModel ==
  A_BN : Inport
  Rate Transition5 : RateTransition  OutPortSampleTime=sensors.starSensor.sampleTime
  Subsystem : Subsystem
  Subsystem Reference{,1..3} (4 alike) : Subsystem  ReferencedSubsystem=starSensorMeasure
  To Workspace1 : ToWorkspace  VariableName=starSensTimeStamp  SaveFormat=Structure With Time  SampleTime=-1
  Zero-Order Hold{,1..3} (4 alike) : ZeroOrderHold  SampleTime=sensors.starSensor.sampleTime
  star mapping : Subsystem
  sMeas1 : Outport
  sMeas2 : Outport  Port=2
  sMeas3 : Outport  Port=3
  sMeas4 : Outport  Port=4
  r1 : Outport  Port=5
  r2 : Outport  Port=6
  r3 : Outport  Port=7
  r4 : Outport  Port=8
  wires:
  Subsystem/1(clock) -> To Workspace1/1
  Subsystem Reference/1 -> sMeas1/1
  Subsystem Reference1/1 -> sMeas2/1
  Subsystem Reference2/1 -> sMeas3/1
  Subsystem Reference3/1 -> sMeas4/1
  A_BN/1 -> Rate Transition5/1
  star mapping/1(s1_N) -> Zero-Order Hold/1, Subsystem Reference/2
  star mapping/2(s2_N) -> Zero-Order Hold1/1, Subsystem Reference1/2
  star mapping/3(s3_N) -> Zero-Order Hold2/1, Subsystem Reference2/2
  star mapping/4(s4_N) -> Zero-Order Hold3/1, Subsystem Reference3/2
  Zero-Order Hold/1 -> r1/1
  Zero-Order Hold3/1 -> r4/1
  Zero-Order Hold2/1 -> r3/1
  Zero-Order Hold1/1 -> r2/1
  Rate Transition5/1 -> star mapping/1(A_BN), Subsystem Reference/1, Subsystem Reference1/1, Subsystem Reference2/1, Subsystem Reference3/1

== system mainModel/thetaOrbit ==
  Constant : Constant  Value=init.theta
  Integrator : Integrator  InitialConditionSource=external  WrapState=on  WrappedStateUpperValue=2*pi  WrappedStateLowerValue=0
  Scope : Scope
  theta_dot : Subsystem
  thetaDot : Outport
  theta : Outport  Port=2
  wires:
  theta_dot/1(theta_dot) -> thetaDot/1, Integrator/1  "theta_dot"
  Constant/1 -> Integrator/2
  Integrator/1 -> theta_dot/1(theta), Scope/1, theta/1  "theta"

== system mainModel/velocityVect ==
  r_N : Inport
  Constant : Constant  Value=3
  Constant1 : Constant  Value=constant.mu
  Constant2 : Constant  Value=init.v0
  Divide : Product  Inputs=*/
  Gain : Gain  Gain=-1
  Integrator1 : Integrator  InitialConditionSource=external
  Power : Math  Operator=pow
  Scope : Scope
  Subsystem Reference : Subsystem  ReferencedSubsystem=vecNorm
  Terminator : Terminator
  v_N : Outport
  wires:
  Constant/1 -> Power/2
  Constant1/1 -> Gain/1
  Power/1 -> Divide/2
  Gain/1 -> Divide/1
  Integrator1/1 -> Scope/1, v_N/1
  Constant2/1 -> Integrator1/2
  r_N/1 -> Subsystem Reference/1
  Subsystem Reference/1 -> Power/1
  Subsystem Reference/2 -> Terminator/1
  Divide/1 -> Integrator1/1

== system mainModel/wHatMatrix ==
  w : Inport
  Constant : Constant  Value=0
  Demux : Demux  Outputs=3
  Gain : Gain  Gain=-1
  Gain1 : Gain  Gain=-1
  Gain2 : Gain  Gain=-1
  Reshape : Reshape  OutputDimensionality=Row vector (2-D)
  Reshape1 : Reshape  OutputDimensionality=Row vector (2-D)
  Reshape2 : Reshape  OutputDimensionality=Row vector (2-D)
  Vector Concatenate : Concatenate  NumInputs=3
  Vector Concatenate1 : Concatenate  NumInputs=3
  Vector Concatenate2 : Concatenate  NumInputs=3
  Vector Concatenate3 : Concatenate  NumInputs=3  Mode=Multidimensional array
  "[w]" : Outport
  wires:
  w/1 -> Demux/1
  Demux/1 -> Vector Concatenate2/2, Gain1/1  "wx"
  Demux/2 -> Gain2/1, Vector Concatenate/3  "wy"
  Demux/3 -> Gain/1, Vector Concatenate1/1  "wz"
  Constant/1 -> Vector Concatenate/1, Vector Concatenate1/2, Vector Concatenate2/3
  Gain/1 -> Vector Concatenate/2
  Gain1/1 -> Vector Concatenate1/3
  Gain2/1 -> Vector Concatenate2/1
  Vector Concatenate1/1 -> Reshape1/1
  Vector Concatenate2/1 -> Reshape2/1
  Vector Concatenate3/1 -> "[w]"/1
  Vector Concatenate/1 -> Reshape/1
  Reshape/1 -> Vector Concatenate3/1
  Reshape2/1 -> Vector Concatenate3/3
  Reshape1/1 -> Vector Concatenate3/2

== system mainModel/DETUMBLING/compute Bdot ==
  B : Inport
  Scope : Scope
  Scope1 : Scope
  Selector : Selector  InputPortWidth=3  IndexOptions=Index vector (dialog)  Indices=1  OutputSizes=1
  Selector1 : Selector  InputPortWidth=3  IndexOptions=Index vector (dialog)  Indices=2  OutputSizes=1
  Selector2 : Selector  InputPortWidth=3  IndexOptions=Index vector (dialog)  Indices=3  OutputSizes=1
  Transfer Fcn1 : TransferFcn  Numerator=[1 0]  Denominator=[1 10]
  Transfer Fcn2 : TransferFcn  Numerator=[1 0]  Denominator=[1 10]
  Transfer Fcn3 : TransferFcn  Numerator=[1 0]  Denominator=[1 10]
  Vector Concatenate : Concatenate  NumInputs=3
  Bdot : Outport
  wires:
  B/1 -> Selector/1, Scope1/1, Selector1/1, Selector2/1
  Selector/1 -> Transfer Fcn3/1
  Selector2/1 -> Transfer Fcn2/1
  Selector1/1 -> Transfer Fcn1/1
  Transfer Fcn3/1 -> Vector Concatenate/1
  Transfer Fcn1/1 -> Vector Concatenate/2
  Transfer Fcn2/1 -> Vector Concatenate/3
  Vector Concatenate/1 -> Scope/1, Bdot/1

== system mainModel/INERTIAL POINTING/Define Error State ==
  qEst : Inport
  wEst : Inport  Port=2
  qTarget : Inport  Port=3
  wTarget : Inport  Port=4
  Gain : Gain  Gain=2
  Minus : Sum  Inputs=+-
  Quaternion Conjugate : aerolibutil/Quaternion Conjugate
  Quaternion Multiplication : aerolibutil/Quaternion Multiplication
  Radians to Degrees : simulink_extras/Transformations/Radians to Degrees
  Reshape : Reshape  OutputDimensionality=Column vector (2-D)
  Reshape1 : Reshape
  Scope : Scope
  Scope1 : Scope
  Selector : Selector  InputPortWidth=4  IndexOptions=Index vector (dialog)  Indices=[2:4]  OutputSizes=1
  To Workspace : ToWorkspace  VariableName=alphaState  SampleTime=-1
  Vector Concatenate : Concatenate
  alphaState : Outport
  wires:
  wTarget/1 -> Minus/1
  wEst/1 -> Minus/2
  Minus/1 -> Reshape/1
  Vector Concatenate/1 -> Reshape1/1, alphaState/1  "alphaState"
  Reshape/1 -> Scope/1, Vector Concatenate/2  "[ alphaDotX   alphaDotY     alphaDotZ ]"
  qEst/1 -> Quaternion Conjugate/1
  Quaternion Conjugate/1 -> Quaternion Multiplication/1
  qTarget/1 -> Quaternion Multiplication/2
  Quaternion Multiplication/1 -> Gain/1  "dq"
  Gain/1 -> Selector/1
  Selector/1 -> Radians to Degrees/1, Vector Concatenate/1  "[ alphaX   alphaY     alphaZ ]"
  Reshape1/1 -> To Workspace/1
  Radians to Degrees/1 -> Scope1/1

== system mainModel/INERTIAL POINTING/PD conroller ==
  alphaState : Inport
  Add : Sum
  Add1 : Sum
  Add2 : Sum
  Gain : Gain  Gain=-control.Kp_x
  Gain1 : Gain  Gain=-control.Kp_y
  Gain2 : Gain  Gain=-control.Kd_x
  Gain3 : Gain  Gain=-control.Kp_z
  Gain4 : Gain  Gain=-control.Kd_y
  Gain5 : Gain  Gain=-control.Kd_z
  Scope : Scope
  Selector : Selector  InputPortWidth=6  IndexOptions=Index vector (dialog)  Indices=[1 4]  OutputSizes=1
  Selector1 : Selector  InputPortWidth=6  IndexOptions=Index vector (dialog)  Indices=[2 5]  OutputSizes=1
  Selector2 : Selector  InputPortWidth=6  IndexOptions=Index vector (dialog)  Indices=3  OutputSizes=1
  Selector3 : Selector  InputPortWidth=6  IndexOptions=Index vector (dialog)  Indices=6  OutputSizes=1
  Selector4 : Selector  InputPortWidth=2  IndexOptions=Index vector (dialog)  Indices=1  OutputSizes=1
  Selector5 : Selector  InputPortWidth=2  IndexOptions=Index vector (dialog)  Indices=2  OutputSizes=1
  Selector6 : Selector  InputPortWidth=2  IndexOptions=Index vector (dialog)  Indices=1  OutputSizes=1
  Selector7 : Selector  InputPortWidth=2  IndexOptions=Index vector (dialog)  Indices=2  OutputSizes=1
  Vector Concatenate : Concatenate  NumInputs=3
  controlTq : Outport
  wires:
  alphaState/1 -> Selector3/1, Selector2/1, Selector1/1, Selector/1
  Selector2/1 -> Gain3/1  "alphaZ"
  Selector3/1 -> Gain5/1  "alphaDotZ"
  Selector1/1 -> Selector6/1, Selector7/1  "[ alphaY    alphaDotY ]"
  Selector/1 -> Selector5/1, Selector4/1  "[ alphaX    alphaDotX ]"
  Selector4/1 -> Gain/1  "alphaX"
  Selector5/1 -> Gain2/1  "alphaDotX"
  Selector6/1 -> Gain1/1  "alphaY"
  Selector7/1 -> Gain4/1  "alphaDotY"
  Gain3/1 -> Add/1
  Gain5/1 -> Add/2
  Add/1 -> Vector Concatenate/3  "zWheelTq"
  Gain2/1 -> Add1/2
  Gain/1 -> Add1/1
  Gain4/1 -> Add2/2
  Gain1/1 -> Add2/1
  Add2/1 -> Vector Concatenate/2  "yMagTq"
  Add1/1 -> Vector Concatenate/1  "xMagTq"
  Vector Concatenate/1 -> Scope/1, controlTq/1  "[ xMAgTq yMagTq   zWheelTq ]"

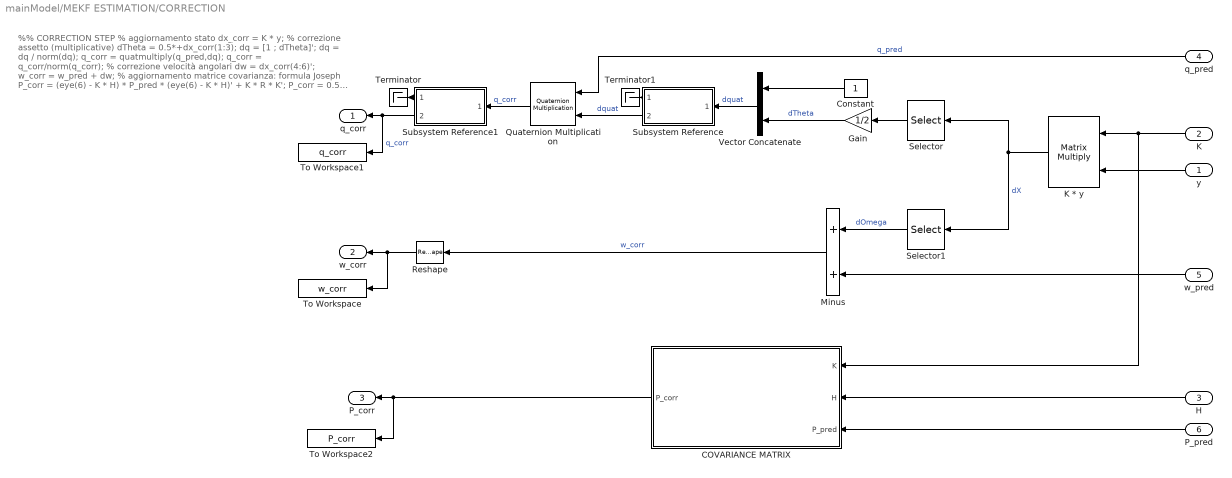
== system mainModel/MEKF ESTIMATION/CORRECTION ==
  note: %% CORRECTION STEP
      | % aggiornamento stato
      | dx_corr = K * y;
      | % correzione assetto (multiplicative)
      | dTheta = 0.5*+dx_corr(1:3);
      | dq = [1 ; dTheta]';
      | dq = dq / norm(dq);
      | q_corr = quatmultiply(q_pred,dq);
      | q_corr = q_corr/norm(q_corr);
      | % correzione velocità angolari
      | dw = dx_corr(4:6)';
      | w_corr = w_pred + dw;
      | % aggiornamento matrice covarianza: formula Joseph
      | P_corr = (eye(6) - K * H) * P_pred * (eye(6) - K * H)' + K * R * K';
      | P_corr = 0.5 * (P_corr + P_corr'); % Simmetria
      | min_cov = 1e-10; % Valore minimo di incertezza
      | for i = 1:6
      | if P_corr(i,i) < min_cov
      | P_corr(i,i) = min_cov;
      | end
      | end
  y : Inport
  K : Inport  Port=2
  H : Inport  Port=3
  q_pred : Inport  Port=4
  w_pred : Inport  Port=5
  P_pred : Inport  Port=6
  COVARIANCE MATRIX : Subsystem
  Constant : Constant
  Gain : Gain  Gain=1/2
  K * y : Product  Multiplication=Matrix(*)
  Minus : Sum
  Quaternion Multiplication : aerolibutil/Quaternion Multiplication
  Reshape : Reshape  OutputDimensionality=Row vector (2-D)
  Selector : Selector  InputPortWidth=6  IndexOptions=Index vector (dialog)  Indices=[1:3]  OutputSizes=1
  Selector1 : Selector  InputPortWidth=6  IndexOptions=Index vector (dialog)  Indices=[4:6]  OutputSizes=1
  Subsystem Reference : Subsystem  ReferencedSubsystem=vecNorm
  Subsystem Reference1 : Subsystem  ReferencedSubsystem=vecNorm
  Terminator : Terminator
  Terminator1 : Terminator
  To Workspace : ToWorkspace  VariableName=w_corr  SampleTime=-1
  To Workspace1 : ToWorkspace  VariableName=q_corr  SampleTime=-1
  To Workspace2 : ToWorkspace  VariableName=P_corr  SampleTime=-1
  Vector Concatenate : Concatenate
  q_corr : Outport
  w_corr : Outport  Port=2
  P_corr : Outport  Port=3
  wires:
  K/1 -> K * y/1, COVARIANCE MATRIX/1(K)
  y/1 -> K * y/2
  K * y/1 -> Selector1/1, Selector/1  "dX"
  Selector/1 -> Gain/1
  Selector1/1 -> Minus/1  "dOmega"
  Gain/1 -> Vector Concatenate/2  "dTheta"
  w_pred/1 -> Minus/2
  Minus/1 -> Reshape/1  "w_corr"
  Constant/1 -> Vector Concatenate/1
  Vector Concatenate/1 -> Subsystem Reference/1  "dquat"
  Subsystem Reference/2 -> Quaternion Multiplication/2  "dquat"
  Subsystem Reference1/2 -> To Workspace1/1, q_corr/1  "q_corr"
  Quaternion Multiplication/1 -> Subsystem Reference1/1  "q_corr"
  Subsystem Reference/1 -> Terminator1/1
  Subsystem Reference1/1 -> Terminator/1
  q_pred/1 -> Quaternion Multiplication/1  "q_pred"
  COVARIANCE MATRIX/1(P_corr) -> To Workspace2/1, P_corr/1
  H/1 -> COVARIANCE MATRIX/2(H)
  P_pred/1 -> COVARIANCE MATRIX/3(P_pred)
  Reshape/1 -> To Workspace/1, w_corr/1

== system mainModel/MEKF ESTIMATION/MEASUREMENT ==
  note: scalar-last2scalar-first
  q_meas_in : Inport
  b_meas_B : Inport  Port=2
  b_real_N : Inport  Port=3
  q_pred : Inport  Port=4
  P_pred : Inport  Port=5
  Constant : Constant  Value=MEKF.R
  Demux : Demux
  KALMAN GAIN : Subsystem
  Mux : Mux
  RESIDUALS : Subsystem
  SENSITIVITY MATRIX : Subsystem
  y : Outport
  K : Outport  Port=2
  H : Outport  Port=3
  wires:
  q_meas_in/1 -> Demux/1
  Demux/2 -> Mux/3
  Mux/1 -> RESIDUALS/1(q_meas)  "q_meas"
  Demux/4 -> Mux/1
  Demux/3 -> Mux/4
  Demux/1 -> Mux/2
  RESIDUALS/1(y) -> y/1
  SENSITIVITY MATRIX/1(H) -> KALMAN GAIN/1(H), H/1
  KALMAN GAIN/1(K) -> K/1
  P_pred/1 -> KALMAN GAIN/2(P_pred)
  Constant/1 -> KALMAN GAIN/3(R)
  q_pred/1 -> RESIDUALS/2(q_pred)
  b_meas_B/1 -> RESIDUALS/3(b_meas_B)
  b_real_N/1 -> RESIDUALS/4(b_real_N)
  RESIDUALS/2(b_pred) -> SENSITIVITY MATRIX/1(b_pred)

== system mainModel/MEKF ESTIMATION/PREDICTION ==
  q_corr : Inport
  w_corr : Inport  Port=2
  P_corr : Inport  Port=3
  J : Inport  Port=4
  distTq : Inport  Port=5
  controlTq : Inport  Port=6
  hWheel : Inport  Port=7
  hDotWheel : Inport  Port=8
  COVARIANCE MATRIX PROPAGATION : Subsystem
  STATE PROPAGATION : Subsystem
  q_pred : Outport
  w_pred : Outport  Port=2
  P_pred : Outport  Port=3
  wires:
  q_corr/1 -> STATE PROPAGATION/1(q_corr)
  w_corr/1 -> STATE PROPAGATION/2(w_corr)
  J/1 -> STATE PROPAGATION/3(J)
  distTq/1 -> STATE PROPAGATION/4(distTq)
  controlTq/1 -> STATE PROPAGATION/5(controlTq)
  hWheel/1 -> STATE PROPAGATION/6(hWheel)
  hDotWheel/1 -> STATE PROPAGATION/7(hDotWheel)
  P_corr/1 -> COVARIANCE MATRIX PROPAGATION/1(P_corr)
  STATE PROPAGATION/1(q_pred) -> q_pred/1
  STATE PROPAGATION/2(w_pred) -> w_pred/1
  COVARIANCE MATRIX PROPAGATION/1(P_pred) -> P_pred/1

== system mainModel/Magnetorquers/Subsystem ==
  controlTq : Inport
  B : Inport  Port=2
  det2point : EnablePort
  Constant : Constant  Value=0
  Cross Product1 : matrix_library/Cross Product
  Divide : Product  Inputs=*/
  Dot Product : DotProduct  OutDataTypeStr=Inherit: Inherit via internal rule
  Saturation : Saturate  UpperLimit=actuators.magTorq.maxDipole  LowerLimit=-actuators.magTorq.maxDipole
  Selector : Selector  InputPortWidth=3  IndexOptions=Index vector (dialog)  Indices=1  OutputSizes=1
  Selector1 : Selector  InputPortWidth=3  IndexOptions=Index vector (dialog)  Indices=2  OutputSizes=1
  Vector Concatenate : Concatenate  NumInputs=3
  m : Outport
  wires:
  Constant/1 -> Vector Concatenate/3
  Selector/1 -> Vector Concatenate/1
  Dot Product/1 -> Divide/2
  Divide/1 -> Saturation/1
  controlTq/1 -> Selector/1, Selector1/1
  Cross Product1/1 -> Divide/1
  Selector1/1 -> Vector Concatenate/2
  B/1 -> Cross Product1/1, Dot Product/1, Dot Product/2
  Saturation/1 -> m/1  "m"
  Vector Concatenate/1 -> Cross Product1/2  "magControlTq"

== system mainModel/TRIAD/angular rates estimation TRIAD  ==
  A_BN_est : Inport
  Discrete Derivative : simulink/Discrete/Discrete Derivative  gainval=1.0  ICPrevScaledInput=0.0  OutMin=[]  OutMax=[]  OutDataType=fixdt(1, 16)  OutScaling=2^-10  DoSatur=off
  Gain : Gain  Gain=-1
  Gain1 : Gain  Gain=1/2
  Gain2 : Gain  Gain=1/2
  Gain3 : Gain  Gain=1/2
  MatrixMultiply : Product  Multiplication=Matrix(*)
  Minus : Sum  Inputs=+-
  Minus1 : Sum  Inputs=+-
  Minus2 : Sum  Inputs=+-
  Selector : Selector  NumberOfDimensions=2  InputPortWidth=3  IndexOptions=Index vector (dialog),Index vector (dialog)  Indices=2,1  OutputSizes=1,1
  Selector1 : Selector  NumberOfDimensions=2  InputPortWidth=3  IndexOptions=Index vector (dialog),Index vector (dialog)  Indices=1,2  OutputSizes=1,1
  Selector2 : Selector  NumberOfDimensions=2  InputPortWidth=3  IndexOptions=Index vector (dialog),Index vector (dialog)  Indices=1,3  OutputSizes=1,1
  Selector3 : Selector  NumberOfDimensions=2  InputPortWidth=3  IndexOptions=Index vector (dialog),Index vector (dialog)  Indices=3,1  OutputSizes=1,1
  Selector5 : Selector  NumberOfDimensions=2  InputPortWidth=3  IndexOptions=Index vector (dialog),Index vector (dialog)  Indices=2,3  OutputSizes=1,1
  Selector6 : Selector  NumberOfDimensions=2  InputPortWidth=3  IndexOptions=Index vector (dialog),Index vector (dialog)  Indices=3,2  OutputSizes=1,1
  Transpose : Math  Operator=transpose
  Vector Concatenate : Concatenate  NumInputs=3
  w_estTRIAD : Outport
  wires:
  A_BN_est/1 -> Discrete Derivative/1, Transpose/1
  Discrete Derivative/1 -> MatrixMultiply/1
  Transpose/1 -> MatrixMultiply/2
  MatrixMultiply/1 -> Gain/1
  Selector/1 -> Minus/1
  Selector1/1 -> Minus/2
  Selector2/1 -> Minus1/1
  Selector3/1 -> Minus1/2
  Selector6/1 -> Minus2/1
  Selector5/1 -> Minus2/2
  Minus/1 -> Gain1/1
  Minus1/1 -> Gain2/1
  Minus2/1 -> Gain3/1
  Vector Concatenate/1 -> w_estTRIAD/1
  Gain1/1 -> Vector Concatenate/1
  Gain2/1 -> Vector Concatenate/2
  Gain3/1 -> Vector Concatenate/3
  Gain/1 -> Selector6/1, Selector5/1, Selector3/1, Selector/1, Selector1/1, Selector2/1

== system mainModel/TRIAD/attitudeDetermination_TRIAD ==
  sMeas1 : Inport
  sMeas2 : Inport  Port=2
  r1 : Inport  Port=3
  r2 : Inport  Port=4
  TRIAD - DCM determination : Subsystem
  To Workspace : ToWorkspace  VariableName=A_BN_TRIAD  SampleTime=-1
  A_BN_est : Outport
  wires:
  TRIAD - DCM determination/1(A_BN_est_TRIAD) -> To Workspace/1, A_BN_est/1
  sMeas1/1 -> TRIAD - DCM determination/1(sMeas1)
  sMeas2/1 -> TRIAD - DCM determination/2(sMeas2)
  r2/1 -> TRIAD - DCM determination/4(r2)
  r1/1 -> TRIAD - DCM determination/3(r1)
